simulink model "simulation"  (R2023b)
settings: Solver=VariableStepAuto  StartTime=0.0  StopTime=1  RelTol=1e-3
values from neighbouring files (symbols this model uses):
  A = [0,   1,   0,     0 ... (first row only)    [design_ss_controller.m]
  B = [0; b21; 0; b41]    [design_ss_controller.m]
  C = [1 0 0 0]    [design_ss_controller.m]
  K1 = -KN(5)    [design_ss_controller.m]
  K2 = KN(1:4)    [design_ss_controller.m]
  T = Tr/10    [design_ss_controller.m]
settings Model: Creator=Celso  LastModifiedBy=Sr. Roque

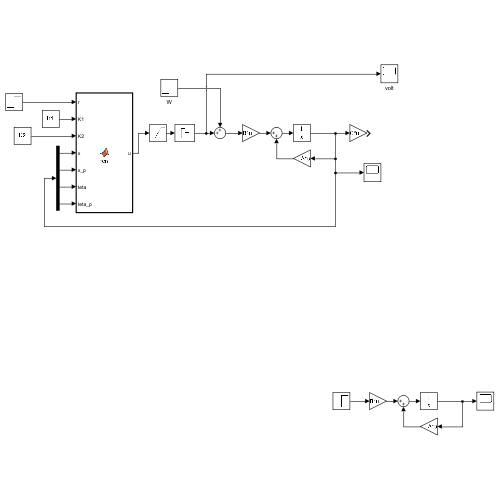
[thumbnail: Simulink's stored preview of the top-level diagram]
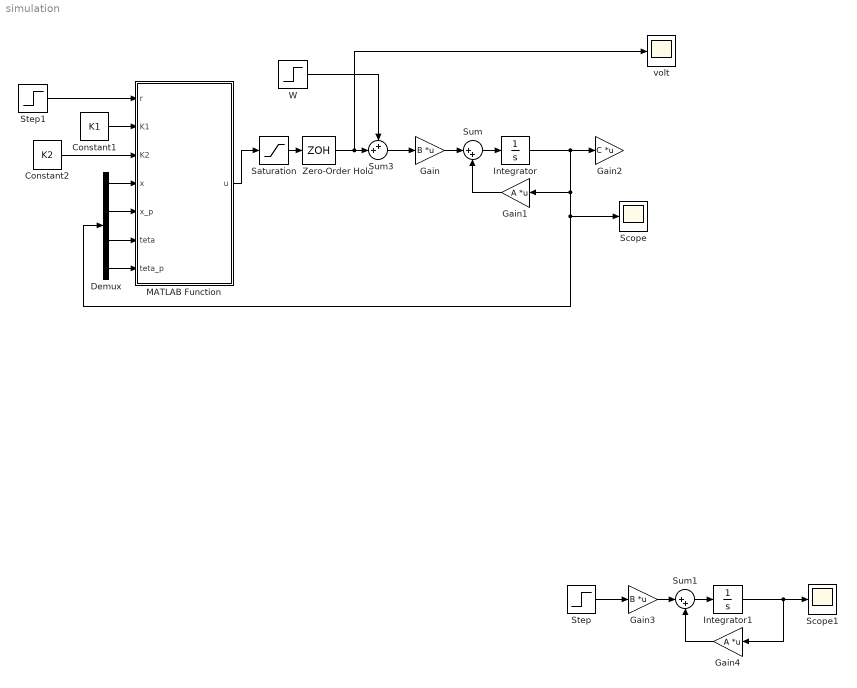
== system simulation ==
  Constant1 : Constant  Value=K1
  Constant2 : Constant  Value=K2
  Demux : Demux
  Gain : Gain  Gain=B  Multiplication=Matrix(K*u)
  Gain1 : Gain  Gain=A  Multiplication=Matrix(K*u)
  Gain2 : Gain  Gain=C  Multiplication=Matrix(K*u)
  Gain3 : Gain  Gain=B  Multiplication=Matrix(K*u)
  Gain4 : Gain  Gain=A  Multiplication=Matrix(K*u)
  Integrator : Integrator  InitialCondition=[0 0 5*pi/180 0]
  Integrator1 : Integrator  InitialCondition=[0 0 1*pi/180 0]
  MATLAB Function : MATLAB Function  TreatAsAtomicUnit=on  SystemSampleTime=T
  Saturation : Saturate  UpperLimit=11  LowerLimit=-11
  Scope : Scope
  Scope1 : Scope
  Step : Step  Time=0  After=0  SampleTime=0
  Step1 : Step  Time=0  After=0  SampleTime=0
  Sum : Sum  Inputs=|++
  Sum1 : Sum  Inputs=|++
  Sum3 : Sum  Inputs=++|
  W : Step  Time=4  After=0  SampleTime=0
  Zero-Order Hold : ZeroOrderHold  SampleTime=T
  volt : Scope
  wires:
  W/1 -> Sum3/1
  Zero-Order Hold/1 -> volt/1, Sum3/2
  MATLAB Function/1(u) -> Saturation/1
  Saturation/1 -> Zero-Order Hold/1
  Sum3/1 -> Gain/1
  Gain/1 -> Sum/1
  Sum/1 -> Integrator/1
  Gain1/1 -> Sum/2
  Integrator/1 -> Gain2/1, Demux/1, Scope/1, Gain1/1
  Step1/1 -> MATLAB Function/1(r)
  Constant1/1 -> MATLAB Function/2(K1)
  Constant2/1 -> MATLAB Function/3(K2)
  Demux/1 -> MATLAB Function/4(x)
  Demux/2 -> MATLAB Function/5(x_p)
  Demux/3 -> MATLAB Function/6(teta)
  Demux/4 -> MATLAB Function/7(teta_p)
  Gain3/1 -> Sum1/1
  Gain4/1 -> Sum1/2
  Sum1/1 -> Integrator1/1
  Integrator1/1 -> Scope1/1, Gain4/1
  Step/1 -> Gain3/1

== matlab function simulation/MATLAB Function ==
  data: r input; K1 input; K2 input; x input; x_p input; teta input; u output; teta_p input
function u = fcn(r,K1,K2, x,x_p,teta,teta_p)

persistent Int;

if isempty(Int),
    Int=0;
end;

e=r-x;
Int = Int + e;  %v(k) = v(k-1) + r-y
u = K1*Int - K2(1)*x - K2(2)*x_p - K2(3)*teta - K2(4)*teta_p;
